simulink model "blueprint"  (R2017b)
settings: Solver=VariableStepAuto  StartTime=0.0  StopTime=10.0  RelTol=1e-3
undefined symbols (not defined in the file or in its folder): genNextCustomer, m, n
libraries: simulink x2
settings Model: Creator=okeee  LastModifiedBy=okeee

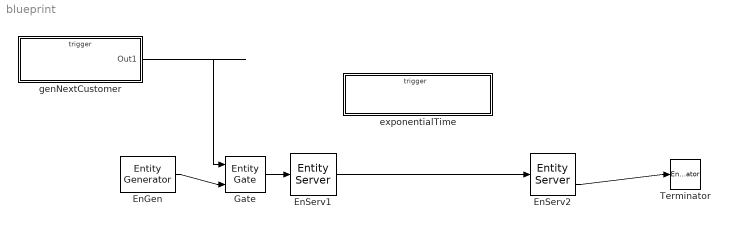
== system blueprint ==
  EnGen : EntityGenerator  OutputPortMessageModes=m  Period=0  GenerateAction=|  AttributeName=lambda|mu|GenTime|ServiceTime  AttributeInitialValue=1|1|1|1  EntityType=Structured  EntityTypeName=Gen
      | entity.GenTime = exponentialTime(entity.lambda);
      | entity.ServiceTime = exponentialTime(entity.mu);
  EnServ1 : EntityServer  InputPortMessageModes=m  OutputPortMessageModes=m  Capacity=1  ServiceTimeSource=Attribute  ServiceTimeAttributeName=GenTime
  EnServ2 : EntityServer  InputPortMessageModes=m  OutputPortMessageModes=n,m  Capacity=1  ServiceTimeSource=Attribute  ServiceTimeAction=|  NumberEntitiesInBlock=on
      | % Exponential service time with rate 1
      | %mean = 1;
      | dt   = exponentialTime(0.3164);
      | disp(dt);
      settings: OutputPortMap=o1,o9
  Gate : EntityGate  InputPortMessageModes=m,m  OutputPortMessageModes=m  OperatingMode=Release gate  OpenGateAtSimulationStart=on
  Terminator : EntityTerminator  InputPortMessageModes=m  EntryAction=genNextCustomer();
  exponentialTime : Subsystem  TreatAsAtomicUnit=on
  genNextCustomer : Subsystem  TreatAsAtomicUnit=on
  wires:
  EnServ1/1 -> EnServ2/1
  EnGen/1 -> Gate/2
  genNextCustomer/1(Out1) -> Gate/1
  Gate/1 -> EnServ1/1
  EnServ2/2 -> Terminator/1

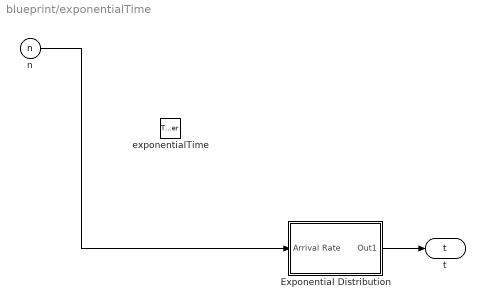
== system blueprint/exponentialTime ==
  exponentialTime : TriggerPort  TriggerType=function-call  IsSimulinkFunction=on  FunctionName=exponentialTime  VariantControl=Variant
  Exponential Distribution : Subsystem
  n : ArgIn  ArgumentName=n
  t : ArgOut  DisableCoverage=on  ArgumentName=t
  wires:
  n/1 -> Exponential Distribution/1(Arrival Rate)
  Exponential Distribution/1(Out1) -> t/1

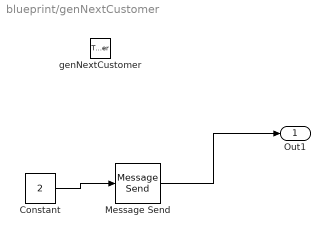
== system blueprint/genNextCustomer ==
  genNextCustomer : TriggerPort  TriggerType=function-call  IsSimulinkFunction=on  FunctionName=genNextCustomer  FunctionVisibility=scoped  VariantControl=Variant
  Constant : Constant  Value=2
  Message Send : MessageSend  OutputPortMessageModes=m
      settings: InputPortMap=u1
  Out1 : Outport
  wires:
  Message Send/1 -> Out1/1
  Constant/1 -> Message Send/1

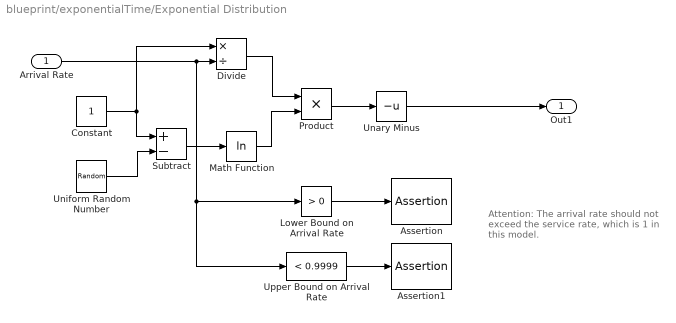
== system blueprint/exponentialTime/Exponential Distribution ==
  note: Attention: The arrival rate
      | should not exceed the service
      | rate, which is 1 in this model.
  Arrival Rate : Inport
  Assertion : Assertion
  Assertion1 : Assertion
  Constant : Constant
  Divide : Product  Inputs=*/
  Lower Bound on Arrival Rate : simulink/Logic and Bit Operations/Compare To Constant  relop=>  const=0  OutDataTypeStr=uint8  ZeroCross=off
  Math Function : Math  Operator=log  SaturateOnIntegerOverflow=on
  Product : Product  RndMeth=Zero
  Subtract : Sum  Inputs=+-
  Unary Minus : UnaryMinus
  Uniform Random Number : UniformRandomNumber  Minimum=0  Seed=rand
  "Upper Bound on Arrival Rate " : simulink/Logic and Bit Operations/Compare To Constant  relop=<  const=0.9999  OutDataTypeStr=uint8  ZeroCross=off
  Out1 : Outport
  wires:
  Arrival Rate/1 -> Divide/2, Lower Bound on Arrival Rate/1, "Upper Bound on Arrival Rate "/1
  Unary Minus/1 -> Out1/1
  Product/1 -> Unary Minus/1
  Math Function/1 -> Product/2
  Divide/1 -> Product/1
  Constant/1 -> Divide/1, Subtract/1
  Uniform Random Number/1 -> Subtract/2
  Lower Bound on Arrival Rate/1 -> Assertion/1
  "Upper Bound on Arrival Rate "/1 -> Assertion1/1
  Subtract/1 -> Math Function/1
